simulink model "someex"  (R2022b)
settings: Solver=VariableStepAuto  StartTime=0.0  StopTime=10.0  RelTol=1e-3
settings Model: Creator=Brigosha_Guest  LastModifiedBy=Brigosha_Guest

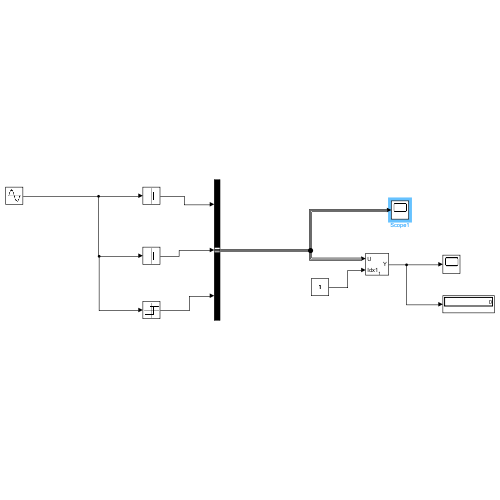
[thumbnail: Simulink's stored preview of the top-level diagram]
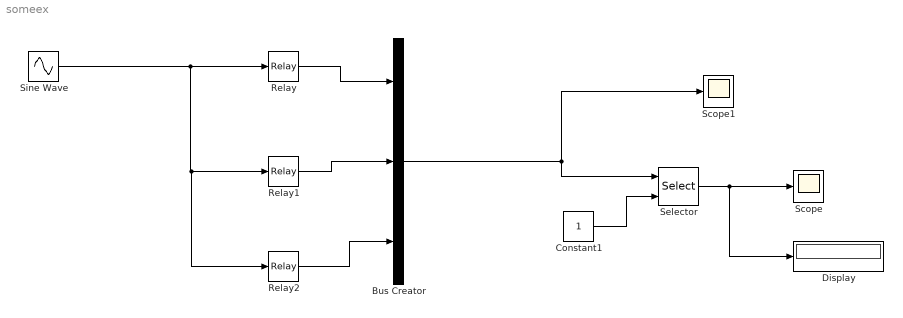
== system someex ==
  Bus Creator : BusCreator  Inputs=3
  Constant1 : Constant
  Display : Display
  Relay : Relay  OnOutputValue=5
  Relay1 : Relay  OnOutputValue=10  OffOutputValue=5
  Relay2 : Relay  OnOutputValue=12  OffOutputValue=10
  Scope : Scope
  Scope1 : Scope
  Selector : Selector  InputPortWidth=3  IndexOptions=Index vector (port)  Indices=[1 3]  OutputSizes=1
  Sine Wave : Sin  Amplitude=24  SampleTime=0
  wires:
  Sine Wave/1 -> Relay2/1, Relay1/1, Relay/1
  Relay/1 -> Bus Creator/1
  Relay1/1 -> Bus Creator/2
  Relay2/1 -> Bus Creator/3
  Bus Creator/1 -> Selector/1, Scope1/1
  Constant1/1 -> Selector/2
  Selector/1 -> Display/1, Scope/1
